simulink model "ICFEMex1"  (R2020a)
settings: Solver=VariableStepAuto  StartTime=0.0  StopTime=10.0  RelTol=1e-3
settings Model: Creator=apple  LastModifiedBy=bzhan
settings DebuggingCC: ArithmeticOperatorsInVariantConditions=warning
settings SFSimCC: CustomCodeUndefinedFunction=UseInterfaceOnly

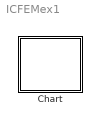
== system ICFEMex1 ==
  Chart : Stateflow chart  TreatAsAtomicUnit=on

== stateflow chart ICFEMex1/Chart ==
  state A
    en: x = 0;
  state B
  (junction 15) -> B : [x>0]
  A -> (junction 15) [order 1] : {fprintf("A");}/{fprintf("B");}
  (default) -> A
  A -> B [order 2] : {x=x+1;fprintf("C");}/{fprintf("D");}
  data: x local
